simulink model "Complete_Model"  (R2015a)
settings: Solver=ode45  StartTime=0.0  StopTime=35  RelTol=1e-4
values from neighbouring files (symbols this model uses):
  g = 9.71    [Run_First.m]
undefined symbols (not defined in the file or in its folder): Earth, Receive, Send, WGS84
libraries: simulink x26, aerolibconvert2 x4, aerolibfltsims x3, aerolib6dof2 x1, aerolibnav x1, aerolibtransform2 x1, aerolibanimutils x1
settings Model: CovSFcnEnable=off  Creator=behill  LastModifiedBy=Bryce
settings DebuggingCC: AlgebraicLoopMsg=none  UnderspecifiedInitializationDetection=Classic  MergeDetectMultiDrivingBlocksExec=none

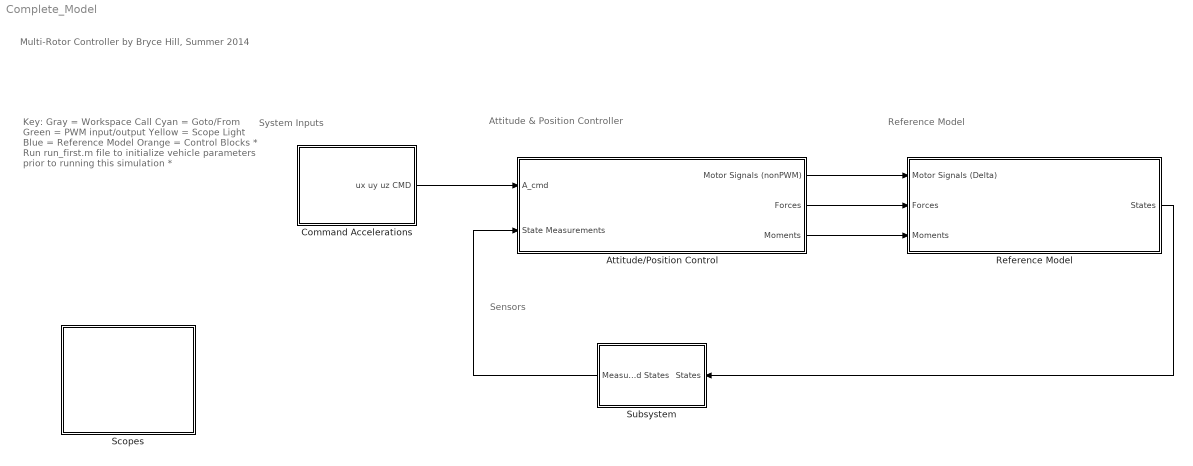
== system Complete_Model ==
  note: Sensors
  note: Reference Model
  note: Attitude & Position Controller
  note: System Inputs
  note: Multi-Rotor Controller
      | by Bryce Hill, Summer 2014
  note: Key:
      | Gray = Workspace Call
      | Cyan = Goto/From
      | Green = PWM input/output
      | Yellow = Scope
      | Light Blue = Reference Model
      | Orange = Control Blocks
      |
      | * Run run_first.m file to initialize vehicle parameters prior to running this simulation *
  Attitude/Position Control : Subsystem
  Command Accelerations : Subsystem
  Reference Model : Subsystem
  Scopes : Subsystem
  Subsystem : Subsystem
  wires:
  Command Accelerations/1(ux uy uz CMD) -> Attitude/Position Control/1(A_cmd)
  Attitude/Position Control/1(Motor Signals (nonPWM)) -> Reference Model/1(Motor Signals (Delta))
  Attitude/Position Control/2(Forces) -> Reference Model/2(Forces)
  Attitude/Position Control/3(Moments) -> Reference Model/3(Moments)
  Reference Model/1(States) -> Subsystem/1(States)
  Subsystem/1(Measured States) -> Attitude/Position Control/2(State Measurements)

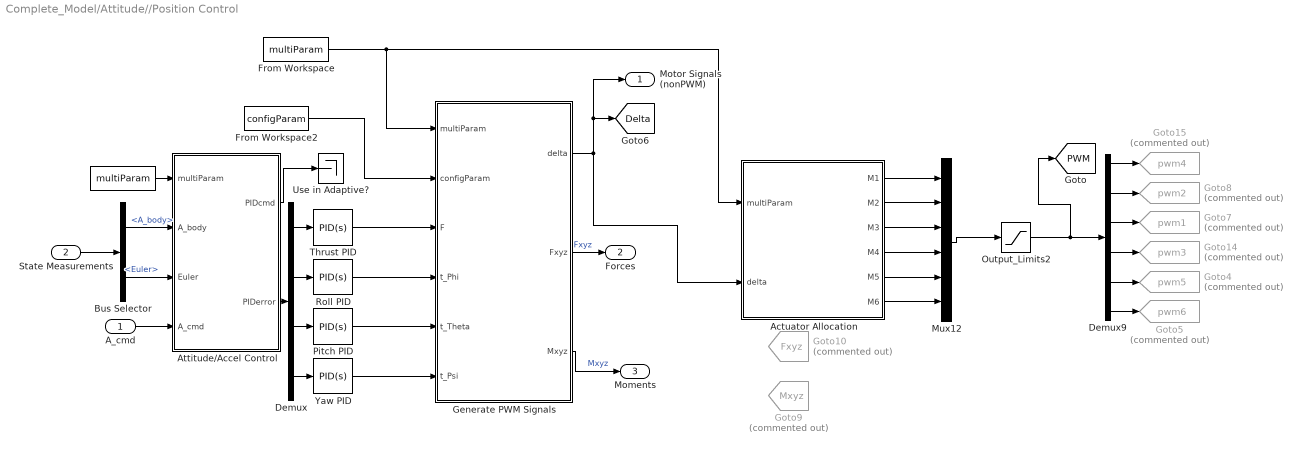
== system Complete_Model/Attitude//Position Control ==
  A_cmd : Inport
  State Measurements : Inport  Port=2
  " " : FromWorkspace  VariableName=multiParam  SampleTime=0
  Actuator Allocation : MATLAB Function  TreatAsAtomicUnit=on
  "Attitude/Accel Control " : MATLAB Function  TreatAsAtomicUnit=on
  Bus Selector : BusSelector  OutputSignals=A_body,Euler
  Demux : Demux
  Demux9 : Demux  Outputs=6
  From Workspace : FromWorkspace  VariableName=multiParam  SampleTime=0
  From Workspace2 : FromWorkspace  VariableName=configParam  SampleTime=0
  Generate PWM Signals : MATLAB Function  TreatAsAtomicUnit=on
  Goto10 : Goto  Commented=on  GotoTag=Fxyz  TagVisibility=global
  Goto14 : Goto  Commented=on  GotoTag=pwm3  TagVisibility=global
  Goto15 : Goto  Commented=on  GotoTag=pwm4  TagVisibility=global
  Goto4 : Goto  Commented=on  GotoTag=pwm5  TagVisibility=global
  Goto5 : Goto  Commented=on  GotoTag=pwm6  TagVisibility=global
  Goto7 : Goto  Commented=on  GotoTag=pwm1  TagVisibility=global
  Goto8 : Goto  Commented=on  GotoTag=pwm2  TagVisibility=global
  Goto9 : Goto  Commented=on  GotoTag=Mxyz  TagVisibility=global
  Mux12 : Mux  Inputs=6
  Output_Limits2 : Saturate  UpperLimit=2000  LowerLimit=1000
  Pitch PID : simulink/Continuous/PID Controller  Controller=PID  TimeDomain=Continuous-time  SampleTime=-1  IntegratorMethod=Forward Euler  FilterMethod=Forward Euler  Form=Parallel  UseFilter=on  ControllerParametersSource=internal  P=0.0917183656646997  I=0.00072113153908676  D=1.05906791895105  N=2.12291335792304  InitialConditionSource=internal  InitialConditionForIntegrator=0  InitialConditionForFilter=0  ExternalReset=none  LimitOutput=off  UpperSaturationLimit=inf  LowerSaturationLimit=-inf  LinearizeAsGain=on  AntiWindupMode=none  Kb=1  TrackingMode=off  Kt=1  PParamMin=[]  PParamMax=[]  IParamMin=[]  IParamMax=[]  DParamMin=[]  DParamMax=[]  NParamMin=[]  NParamMax=[]  KbParamMin=[]  KbParamMax=[]  KtParamMin=[]  KtParamMax=[]  POutMin=[]  POutMax=[]  IOutMin=[]  IOutMax=[]  DOutMin=[]  DOutMax=[]  NOutMin=[]  NOutMax=[]  KbOutMin=[]  KbOutMax=[]  KtOutMin=[]  KtOutMax=[]  IntegratorOutMin=[]  IntegratorOutMax=[]  FilterOutMin=[]  FilterOutMax=[]  SumOutMin=[]  SumOutMax=[]  SumI1OutMin=[]  SumI1OutMax=[]  SumI2OutMin=[]  SumI2OutMax=[]  SumI3OutMin=[]  SumI3OutMax=[]  SumDOutMin=[]  SumDOutMax=[]  SaturationOutMin=[]  SaturationOutMax=[]  IntegratorContinuousStateAttributes=''  IntegratorStateMustResolveToSignalObject=off  IntegratorRTWStateStorageClass=Auto  FilterContinuousStateAttributes=''  FilterStateMustResolveToSignalObject=off  FilterRTWStateStorageClass=Auto  DifferentiatorICPrevScaledInput=0  DifferentiatorOutMin=[]  DifferentiatorOutMax=[]
  Roll PID : simulink/Continuous/PID Controller  Controller=PID  TimeDomain=Continuous-time  SampleTime=-1  IntegratorMethod=Forward Euler  FilterMethod=Forward Euler  Form=Parallel  UseFilter=on  ControllerParametersSource=internal  P=0.231481505773178  I=0.0144568768471083  D=0.336499020225336  N=16.862900200716  InitialConditionSource=internal  InitialConditionForIntegrator=0  InitialConditionForFilter=0  ExternalReset=none  LimitOutput=off  UpperSaturationLimit=inf  LowerSaturationLimit=-inf  LinearizeAsGain=on  AntiWindupMode=none  Kb=1  TrackingMode=off  Kt=1  PParamMin=[]  PParamMax=[]  IParamMin=[]  IParamMax=[]  DParamMin=[]  DParamMax=[]  NParamMin=[]  NParamMax=[]  KbParamMin=[]  KbParamMax=[]  KtParamMin=[]  KtParamMax=[]  POutMin=[]  POutMax=[]  IOutMin=[]  IOutMax=[]  DOutMin=[]  DOutMax=[]  NOutMin=[]  NOutMax=[]  KbOutMin=[]  KbOutMax=[]  KtOutMin=[]  KtOutMax=[]  IntegratorOutMin=[]  IntegratorOutMax=[]  FilterOutMin=[]  FilterOutMax=[]  SumOutMin=[]  SumOutMax=[]  SumI1OutMin=[]  SumI1OutMax=[]  SumI2OutMin=[]  SumI2OutMax=[]  SumI3OutMin=[]  SumI3OutMax=[]  SumDOutMin=[]  SumDOutMax=[]  SaturationOutMin=[]  SaturationOutMax=[]  IntegratorContinuousStateAttributes=''  IntegratorStateMustResolveToSignalObject=off  IntegratorRTWStateStorageClass=Auto  FilterContinuousStateAttributes=''  FilterStateMustResolveToSignalObject=off  FilterRTWStateStorageClass=Auto  DifferentiatorICPrevScaledInput=0  DifferentiatorOutMin=[]  DifferentiatorOutMax=[]
  Thrust PID : simulink/Continuous/PID Controller  Controller=PID  TimeDomain=Continuous-time  SampleTime=-1  IntegratorMethod=Forward Euler  FilterMethod=Forward Euler  Form=Parallel  UseFilter=on  ControllerParametersSource=internal  P=10  I=10  D=15  N=100  InitialConditionSource=internal  InitialConditionForIntegrator=0  InitialConditionForFilter=0  ExternalReset=none  LimitOutput=off  UpperSaturationLimit=inf  LowerSaturationLimit=-inf  LinearizeAsGain=on  AntiWindupMode=none  Kb=1  TrackingMode=off  Kt=1  PParamMin=[]  PParamMax=[]  IParamMin=[]  IParamMax=[]  DParamMin=[]  DParamMax=[]  NParamMin=[]  NParamMax=[]  KbParamMin=[]  KbParamMax=[]  KtParamMin=[]  KtParamMax=[]  POutMin=[]  POutMax=[]  IOutMin=[]  IOutMax=[]  DOutMin=[]  DOutMax=[]  NOutMin=[]  NOutMax=[]  KbOutMin=[]  KbOutMax=[]  KtOutMin=[]  KtOutMax=[]  IntegratorOutMin=[]  IntegratorOutMax=[]  FilterOutMin=[]  FilterOutMax=[]  SumOutMin=[]  SumOutMax=[]  SumI1OutMin=[]  SumI1OutMax=[]  SumI2OutMin=[]  SumI2OutMax=[]  SumI3OutMin=[]  SumI3OutMax=[]  SumDOutMin=[]  SumDOutMax=[]  SaturationOutMin=[]  SaturationOutMax=[]  IntegratorContinuousStateAttributes=''  IntegratorStateMustResolveToSignalObject=off  IntegratorRTWStateStorageClass=Auto  FilterContinuousStateAttributes=''  FilterStateMustResolveToSignalObject=off  FilterRTWStateStorageClass=Auto  DifferentiatorICPrevScaledInput=0  DifferentiatorOutMin=[]  DifferentiatorOutMax=[]
  Use in Adaptive? : Terminator
  Yaw PID : simulink/Continuous/PID Controller  Controller=PID  TimeDomain=Continuous-time  SampleTime=-1  IntegratorMethod=Forward Euler  FilterMethod=Forward Euler  Form=Parallel  UseFilter=on  ControllerParametersSource=internal  P=0.00458591828325413  I=3.60565769544884e-05  D=0.0529533959477758  N=2.12291335792304  InitialConditionSource=internal  InitialConditionForIntegrator=0  InitialConditionForFilter=0  ExternalReset=none  LimitOutput=off  UpperSaturationLimit=inf  LowerSaturationLimit=-inf  LinearizeAsGain=on  AntiWindupMode=none  Kb=1  TrackingMode=off  Kt=1  PParamMin=[]  PParamMax=[]  IParamMin=[]  IParamMax=[]  DParamMin=[]  DParamMax=[]  NParamMin=[]  NParamMax=[]  KbParamMin=[]  KbParamMax=[]  KtParamMin=[]  KtParamMax=[]  POutMin=[]  POutMax=[]  IOutMin=[]  IOutMax=[]  DOutMin=[]  DOutMax=[]  NOutMin=[]  NOutMax=[]  KbOutMin=[]  KbOutMax=[]  KtOutMin=[]  KtOutMax=[]  IntegratorOutMin=[]  IntegratorOutMax=[]  FilterOutMin=[]  FilterOutMax=[]  SumOutMin=[]  SumOutMax=[]  SumI1OutMin=[]  SumI1OutMax=[]  SumI2OutMin=[]  SumI2OutMax=[]  SumI3OutMin=[]  SumI3OutMax=[]  SumDOutMin=[]  SumDOutMax=[]  SaturationOutMin=[]  SaturationOutMax=[]  IntegratorContinuousStateAttributes=''  IntegratorStateMustResolveToSignalObject=off  IntegratorRTWStateStorageClass=Auto  FilterContinuousStateAttributes=''  FilterStateMustResolveToSignalObject=off  FilterRTWStateStorageClass=Auto  DifferentiatorICPrevScaledInput=0  DifferentiatorOutMin=[]  DifferentiatorOutMax=[]
  Motor Signals (nonPWM) : Outport
  Forces : Outport  Port=2
  Moments : Outport  Port=3
  tag scope: Delta=global, PWM=global
  wires:
  Yaw PID/1 -> Generate PWM Signals/6(t_Psi)
  Thrust PID/1 -> Generate PWM Signals/3(F)
  Pitch PID/1 -> Generate PWM Signals/5(t_Theta)
  Roll PID/1 -> Generate PWM Signals/4(t_Phi)
  " "/1 -> "Attitude/Accel Control "/1(multiParam)
  "Attitude/Accel Control "/1(PIDcmd) -> Use in Adaptive?/1
  "Attitude/Accel Control "/2(PIDerror) -> Demux/1
  Demux/1 -> Thrust PID/1
  Actuator Allocation/4(M4) -> Mux12/4
  Demux9/5 -> Goto4/1
  Demux9/6 -> Goto5/1
  Actuator Allocation/3(M3) -> Mux12/3
  Actuator Allocation/1(M1) -> Mux12/1
  Demux9/1 -> Goto15/1
  Demux9/2 -> Goto8/1
  Demux9/3 -> Goto7/1
  Demux9/4 -> Goto14/1
  Mux12/1 -> Output_Limits2/1
  Demux/2 -> Roll PID/1
  Demux/4 -> Yaw PID/1
  Generate PWM Signals/1(delta) -> [Delta], Motor Signals (nonPWM)/1, Actuator Allocation/2(delta)
  Demux/3 -> Pitch PID/1
  Actuator Allocation/2(M2) -> Mux12/2
  Generate PWM Signals/2(Fxyz) -> Forces/1  "Fxyz"
  A_cmd/1 -> "Attitude/Accel Control "/4(A_cmd)
  Generate PWM Signals/3(Mxyz) -> Moments/1  "Mxyz"
  Bus Selector/1 -> "Attitude/Accel Control "/2(A_body)  "<A_body>"
  Bus Selector/2 -> "Attitude/Accel Control "/3(Euler)  "<Euler>"
  State Measurements/1 -> Bus Selector/1
  From Workspace/1 -> Actuator Allocation/1(multiParam), Generate PWM Signals/1(multiParam)
  From Workspace2/1 -> Generate PWM Signals/2(configParam)
  Output_Limits2/1 -> Demux9/1, [PWM]
  Actuator Allocation/5(M5) -> Mux12/5
  Actuator Allocation/6(M6) -> Mux12/6

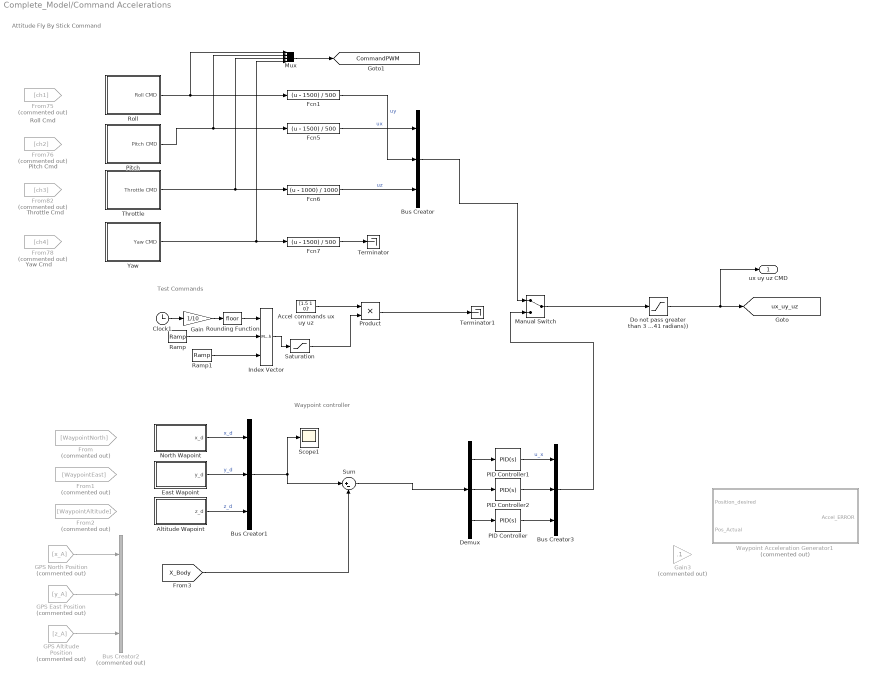
== system Complete_Model/Command Accelerations ==
  note: Waypoint controller
  note: Test Commands
  note: Attitude Fly By Stick Command
  note: Roll Cmd
  note: Throttle Cmd
  note: Yaw Cmd
  note: Pitch Cmd
  Accel commands ux uy uz : Constant  Value=[1.5 1 0]'
  Altitude Wapoint : Subsystem
  Bus Creator : BusCreator  Inputs=3
  Bus Creator1 : BusCreator  Inputs=3
  Bus Creator2 : BusCreator  Commented=on  Inputs=3
  Bus Creator3 : BusCreator  Inputs=3
  Clock1 : Clock
  Demux : Demux  Outputs=3
  Do not pass greater than 3 m/s (23 degrees (.41 radians)) : Saturate  UpperLimit=1  LowerLimit=-1
  East Wapoint : Subsystem
  Fcn1 : Fcn  Expr=(u - 1500) / 500
  Fcn5 : Fcn  Expr=(u - 1500) / 500
  Fcn6 : Fcn  Expr=(u - 1000) / 1000
  Fcn7 : Fcn  Expr=(u - 1500) / 500
  From : From  Commented=on  GotoTag=WaypointNorth
  From1 : From  Commented=on  GotoTag=WaypointEast
  From2 : From  Commented=on  GotoTag=WaypointAltitude
  From75 : From  Commented=on  GotoTag=ch1
  From76 : From  Commented=on  GotoTag=ch2
  From78 : From  Commented=on  GotoTag=ch4
  From82 : From  Commented=on  GotoTag=ch3
  GPS Altitude Position : From  Commented=on  GotoTag=z_A
  GPS East Position : From  Commented=on  GotoTag=y_A
  GPS North Position : From  Commented=on  GotoTag=x_A
  Gain : Gain  Gain=1/10
  Gain3 : Gain  Commented=on  Gain=.1
  Index Vector : MultiPortSwitch  DataPortOrder=Zero-based contiguous  Inputs=2  DiagnosticForDefault=None  zeroidx=on
  Manual Switch : ManualSwitch
  Mux : Mux
  North Wapoint : Subsystem
  PID Controller : simulink/Continuous/PID Controller  Controller=PID  TimeDomain=Continuous-time  SampleTime=-1  IntegratorMethod=Forward Euler  FilterMethod=Forward Euler  Form=Parallel  UseFilter=on  ControllerParametersSource=internal  P=0.00117950118646568  I=9.51975576620891e-07  D=0.104202467385276  N=0.212291335792304  InitialConditionSource=internal  InitialConditionForIntegrator=0  InitialConditionForFilter=0  ExternalReset=none  LimitOutput=off  UpperSaturationLimit=inf  LowerSaturationLimit=-inf  LinearizeAsGain=on  AntiWindupMode=none  Kb=1  TrackingMode=off  Kt=1  PParamMin=[]  PParamMax=[]  IParamMin=[]  IParamMax=[]  DParamMin=[]  DParamMax=[]  NParamMin=[]  NParamMax=[]  KbParamMin=[]  KbParamMax=[]  KtParamMin=[]  KtParamMax=[]  POutMin=[]  POutMax=[]  IOutMin=[]  IOutMax=[]  DOutMin=[]  DOutMax=[]  NOutMin=[]  NOutMax=[]  KbOutMin=[]  KbOutMax=[]  KtOutMin=[]  KtOutMax=[]  IntegratorOutMin=[]  IntegratorOutMax=[]  FilterOutMin=[]  FilterOutMax=[]  SumOutMin=[]  SumOutMax=[]  SumI1OutMin=[]  SumI1OutMax=[]  SumI2OutMin=[]  SumI2OutMax=[]  SumI3OutMin=[]  SumI3OutMax=[]  SumDOutMin=[]  SumDOutMax=[]  SaturationOutMin=[]  SaturationOutMax=[]  IntegratorContinuousStateAttributes=''  IntegratorStateMustResolveToSignalObject=off  IntegratorRTWStateStorageClass=Auto  FilterContinuousStateAttributes=''  FilterStateMustResolveToSignalObject=off  FilterRTWStateStorageClass=Auto  DifferentiatorICPrevScaledInput=0  DifferentiatorOutMin=[]  DifferentiatorOutMax=[]
  PID Controller1 : simulink/Continuous/PID Controller  Controller=PID  TimeDomain=Continuous-time  SampleTime=-1  IntegratorMethod=Forward Euler  FilterMethod=Forward Euler  Form=Parallel  UseFilter=on  ControllerParametersSource=internal  P=8.76810575019982e-09  I=2.11533755573293e-14  D=0.000329957020406041  N=0.000651400313625064  InitialConditionSource=internal  InitialConditionForIntegrator=0  InitialConditionForFilter=0  ExternalReset=none  LimitOutput=off  UpperSaturationLimit=inf  LowerSaturationLimit=-inf  LinearizeAsGain=on  AntiWindupMode=none  Kb=1  TrackingMode=off  Kt=1  PParamMin=[]  PParamMax=[]  IParamMin=[]  IParamMax=[]  DParamMin=[]  DParamMax=[]  NParamMin=[]  NParamMax=[]  KbParamMin=[]  KbParamMax=[]  KtParamMin=[]  KtParamMax=[]  POutMin=[]  POutMax=[]  IOutMin=[]  IOutMax=[]  DOutMin=[]  DOutMax=[]  NOutMin=[]  NOutMax=[]  KbOutMin=[]  KbOutMax=[]  KtOutMin=[]  KtOutMax=[]  IntegratorOutMin=[]  IntegratorOutMax=[]  FilterOutMin=[]  FilterOutMax=[]  SumOutMin=[]  SumOutMax=[]  SumI1OutMin=[]  SumI1OutMax=[]  SumI2OutMin=[]  SumI2OutMax=[]  SumI3OutMin=[]  SumI3OutMax=[]  SumDOutMin=[]  SumDOutMax=[]  SaturationOutMin=[]  SaturationOutMax=[]  IntegratorContinuousStateAttributes=''  IntegratorStateMustResolveToSignalObject=off  IntegratorRTWStateStorageClass=Auto  FilterContinuousStateAttributes=''  FilterStateMustResolveToSignalObject=off  FilterRTWStateStorageClass=Auto  DifferentiatorICPrevScaledInput=0  DifferentiatorOutMin=[]  DifferentiatorOutMax=[]
  PID Controller2 : simulink/Continuous/PID Controller  Controller=PID  TimeDomain=Continuous-time  SampleTime=-1  IntegratorMethod=Forward Euler  FilterMethod=Forward Euler  Form=Parallel  UseFilter=on  ControllerParametersSource=internal  P=0.345806907293553  I=0.007128817123713  D=3.36644459456349  N=372.899120284162  InitialConditionSource=internal  InitialConditionForIntegrator=0  InitialConditionForFilter=0  ExternalReset=none  LimitOutput=off  UpperSaturationLimit=inf  LowerSaturationLimit=-inf  LinearizeAsGain=on  AntiWindupMode=none  Kb=1  TrackingMode=off  Kt=1  PParamMin=[]  PParamMax=[]  IParamMin=[]  IParamMax=[]  DParamMin=[]  DParamMax=[]  NParamMin=[]  NParamMax=[]  KbParamMin=[]  KbParamMax=[]  KtParamMin=[]  KtParamMax=[]  POutMin=[]  POutMax=[]  IOutMin=[]  IOutMax=[]  DOutMin=[]  DOutMax=[]  NOutMin=[]  NOutMax=[]  KbOutMin=[]  KbOutMax=[]  KtOutMin=[]  KtOutMax=[]  IntegratorOutMin=[]  IntegratorOutMax=[]  FilterOutMin=[]  FilterOutMax=[]  SumOutMin=[]  SumOutMax=[]  SumI1OutMin=[]  SumI1OutMax=[]  SumI2OutMin=[]  SumI2OutMax=[]  SumI3OutMin=[]  SumI3OutMax=[]  SumDOutMin=[]  SumDOutMax=[]  SaturationOutMin=[]  SaturationOutMax=[]  IntegratorContinuousStateAttributes=''  IntegratorStateMustResolveToSignalObject=off  IntegratorRTWStateStorageClass=Auto  FilterContinuousStateAttributes=''  FilterStateMustResolveToSignalObject=off  FilterRTWStateStorageClass=Auto  DifferentiatorICPrevScaledInput=0  DifferentiatorOutMin=[]  DifferentiatorOutMax=[]
  Pitch : Subsystem
  Product : Product
  Ramp : simulink/Sources/Ramp  slope=5/5  start=0  X0=0
  Ramp1 : simulink/Sources/Ramp  slope=-2  start=10  X0=5
  Roll : Subsystem
  Rounding Function : Rounding
  Saturation : Saturate  UpperLimit=5  LowerLimit=-5
  Scope1 : Scope
      settings: ShowLegends=on  YMin=0  YMax=10  SaveName=ScopeData8
  Sum : Sum  Inputs=|+-
  Terminator : Terminator
  Terminator1 : Terminator
  Throttle : Subsystem
  Waypoint Acceleration Generator1 : MATLAB Function  Commented=on  TreatAsAtomicUnit=on
  Yaw : Subsystem
  ux uy uz CMD : Outport
  tag scope: CommandPWM=global, ux_uy_uz=global
  wires:
  Fcn7/1 -> Terminator/1
  Mux/1 -> [CommandPWM]
  Fcn6/1 -> Bus Creator/3  "uz"
  Fcn5/1 -> Bus Creator/1  "ux"
  Fcn1/1 -> Bus Creator/2  "uy"
  Bus Creator/1 -> Manual Switch/1
  Roll/1(Roll CMD) -> Mux/1, Fcn1/1
  Pitch/1(Pitch CMD) -> Mux/2, Fcn5/1
  Yaw/1(Yaw CMD) -> Mux/4, Fcn7/1
  Throttle/1(Throttle CMD) -> Fcn6/1, Mux/3
  Saturation/1 -> Product/2
  Rounding Function/1 -> Index Vector/1
  Product/1 -> Terminator1/1
  Accel commands ux uy uz/1 -> Product/1
  Ramp1/1 -> Index Vector/3
  Ramp/1 -> Index Vector/2
  Clock1/1 -> Gain/1
  Index Vector/1 -> Saturation/1
  Gain/1 -> Rounding Function/1
  Manual Switch/1 -> Do not pass greater than 3 m/s (23 degrees (.41 radians))/1
  Do not pass greater than 3 m/s (23 degrees (.41 radians))/1 -> ux uy uz CMD/1, [ux_uy_uz]
  North Wapoint/1(x_d) -> Bus Creator1/1  "x_d"
  East Wapoint/1(y_d) -> Bus Creator1/2  "y_d"
  Altitude Wapoint/1(z_d) -> Bus Creator1/3  "z_d"
  Bus Creator1/1 -> Sum/1, Scope1/1
  [X_Body] -> Sum/2
  GPS North Position/1 -> Bus Creator2/1
  GPS East Position/1 -> Bus Creator2/2
  GPS Altitude Position/1 -> Bus Creator2/3
  Sum/1 -> Demux/1
  Demux/2 -> PID Controller2/1
  PID Controller1/1 -> Bus Creator3/1  "u_x"
  Bus Creator3/1 -> Manual Switch/2
  Demux/3 -> PID Controller/1
  PID Controller/1 -> Bus Creator3/3
  Demux/1 -> PID Controller1/1
  PID Controller2/1 -> Bus Creator3/2

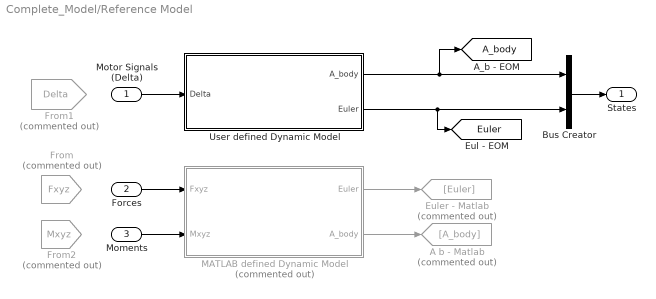
== system Complete_Model/Reference Model ==
  Motor Signals (Delta) : Inport
  Forces : Inport  Port=2
  Moments : Inport  Port=3
  A b - Matlab : Goto  Commented=on  GotoTag=A_body
  Bus Creator : BusCreator  Inputs=2
  Euler - Matlab : Goto  Commented=on  GotoTag=Euler
  From : From  Commented=on  GotoTag=Fxyz  TagVisibility=global
  From1 : From  Commented=on  GotoTag=Delta  TagVisibility=global
  From2 : From  Commented=on  GotoTag=Mxyz  TagVisibility=global
  MATLAB defined Dynamic Model : Subsystem  Commented=on
  User defined Dynamic Model : Subsystem
  States : Outport
  tag scope: A_body=global, Euler=global
  wires:
  MATLAB defined Dynamic Model/1(Euler) -> Euler - Matlab/1
  MATLAB defined Dynamic Model/2(A_body) -> A b - Matlab/1
  Motor Signals (Delta)/1 -> User defined Dynamic Model/1(Delta)
  Forces/1 -> MATLAB defined Dynamic Model/1(Fxyz)
  Moments/1 -> MATLAB defined Dynamic Model/2(Mxyz)
  User defined Dynamic Model/1(A_body) -> [A_body], Bus Creator/1
  User defined Dynamic Model/2(Euler) -> Bus Creator/2, [Euler]
  Bus Creator/1 -> States/1

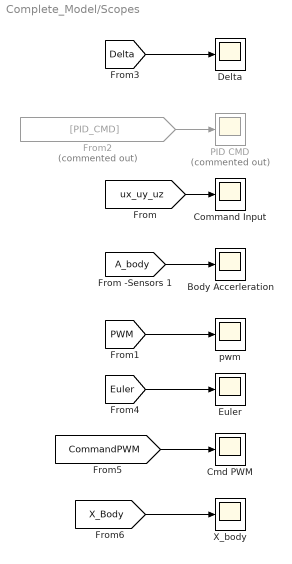
== system Complete_Model/Scopes ==
  Body Accerleration : Scope
      settings: ShowLegends=on  YMin=-1.3  YMax=0.7  SaveName=ScopeData2
  Cmd PWM : Scope
      settings: TimeRange=35  YMin=1500  YMax=1521  SaveName=ScopeData4
  Command Input : Scope
      settings: ShowLegends=on  YMin=-0.25  YMax=0.2  SaveName=ScopeData3
  Delta : Scope
      settings: YMin=27.5  YMax=33
  Euler : Scope
      settings: YMin=-2.75e-07  YMax=2.5e-08  SaveName=ScopeData6
  From2 : From  Commented=on  GotoTag=PID_CMD
  PID CMD : Scope  Commented=on
  X_body : Scope
      settings: ShowLegends=on  YMin=-10  YMax=190  SaveName=ScopeData9
  pwm : Scope
      settings: YMin=1463  YMax=1479  SaveName=ScopeData5
  wires:
  [ux_uy_uz] -> Command Input/1
  [PWM] -> pwm/1
  [A_body] -> Body Accerleration/1
  [Delta] -> Delta/1
  From2/1 -> PID CMD/1
  [Euler] -> Euler/1
  [CommandPWM] -> Cmd PWM/1
  [X_Body] -> X_body/1

== system Complete_Model/Subsystem ==
  States : Inport
  Measured States : Outport
  wires:
  States/1 -> Measured States/1

== system Complete_Model/Command Accelerations/Altitude Wapoint ==
  Clock : Clock
  Constant : Constant  Value=-10
  Constant1 : Constant  Value=10
  Switch : Switch  Criteria=u2 > Threshold  Threshold=30
  z_d : Outport
  wires:
  Clock/1 -> Switch/2
  Constant1/1 -> Switch/3
  Constant/1 -> z_d/1

== system Complete_Model/Command Accelerations/East Wapoint ==
  Clock : Clock
  Constant : Constant  Value=0
  Constant1 : Constant  Value=.01
  Switch : Switch  Criteria=u2 > Threshold  Threshold=30
  y_d : Outport
  wires:
  Clock/1 -> Switch/2
  Constant1/1 -> Switch/3
  Constant/1 -> y_d/1

== system Complete_Model/Command Accelerations/North Wapoint ==
  Clock : Clock
  Constant : Constant  Value=10
  Constant1 : Constant  Value=5
  Switch : Switch  Criteria=u2 > Threshold  Threshold=30
  x_d : Outport
  wires:
  Clock/1 -> Switch/2
  Constant1/1 -> Switch/3
  Constant/1 -> x_d/1

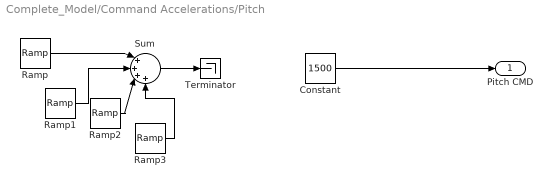
== system Complete_Model/Command Accelerations/Pitch ==
  Constant : Constant  Value=1500
  Ramp : simulink/Sources/Ramp  slope=10  start=5  X0=250
  Ramp1 : simulink/Sources/Ramp  slope=-10  start=10  X0=300
  Ramp2 : simulink/Sources/Ramp  slope=-10  start=15  X0=300
  Ramp3 : simulink/Sources/Ramp  slope=10  start=20  X0=250
  Sum : Sum  Inputs=|++++
  Terminator : Terminator
  Pitch CMD : Outport
  wires:
  Ramp/1 -> Sum/1
  Ramp1/1 -> Sum/2
  Ramp2/1 -> Sum/3
  Ramp3/1 -> Sum/4
  Sum/1 -> Terminator/1
  Constant/1 -> Pitch CMD/1

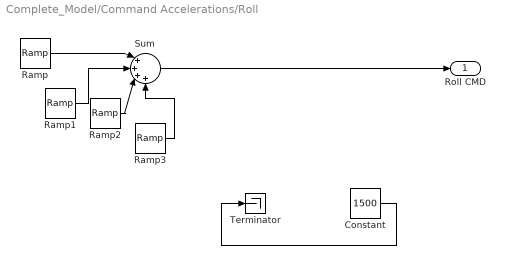
== system Complete_Model/Command Accelerations/Roll ==
  Constant : Constant  Value=1500
  Ramp : simulink/Sources/Ramp  slope=10  start=5  X0=350
  Ramp1 : simulink/Sources/Ramp  slope=-10  start=10  X0=400
  Ramp2 : simulink/Sources/Ramp  slope=-10  start=15  X0=400
  Ramp3 : simulink/Sources/Ramp  slope=10  start=20  X0=350
  Sum : Sum  Inputs=|++++
  Terminator : Terminator
  Roll CMD : Outport
  wires:
  Ramp/1 -> Sum/1
  Ramp1/1 -> Sum/2
  Ramp2/1 -> Sum/3
  Ramp3/1 -> Sum/4
  Constant/1 -> Terminator/1
  Sum/1 -> Roll CMD/1

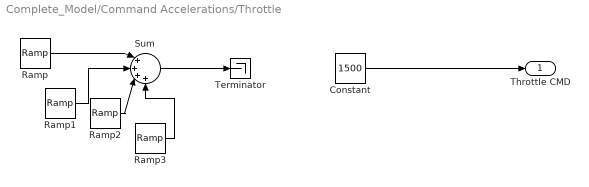
== system Complete_Model/Command Accelerations/Throttle ==
  Constant : Constant  Value=1500
  Ramp : simulink/Sources/Ramp  slope=10  start=5  X0=250
  Ramp1 : simulink/Sources/Ramp  slope=-10  start=10  X0=300
  Ramp2 : simulink/Sources/Ramp  slope=-10  start=15  X0=300
  Ramp3 : simulink/Sources/Ramp  slope=10  start=20  X0=250
  Sum : Sum  Inputs=|++++
  Terminator : Terminator
  Throttle CMD : Outport
  wires:
  Ramp/1 -> Sum/1
  Ramp1/1 -> Sum/2
  Ramp2/1 -> Sum/3
  Ramp3/1 -> Sum/4
  Sum/1 -> Terminator/1
  Constant/1 -> Throttle CMD/1

== system Complete_Model/Command Accelerations/Yaw ==
  Constant : Constant  Value=1500
  Ramp : simulink/Sources/Ramp  slope=10  start=5  X0=250
  Ramp1 : simulink/Sources/Ramp  slope=-10  start=10  X0=300
  Ramp2 : simulink/Sources/Ramp  slope=-10  start=15  X0=300
  Ramp3 : simulink/Sources/Ramp  slope=10  start=20  X0=250
  Sum : Sum  Inputs=|++++
  Terminator : Terminator
  Yaw CMD : Outport
  wires:
  Ramp/1 -> Sum/1
  Ramp1/1 -> Sum/2
  Ramp2/1 -> Sum/3
  Ramp3/1 -> Sum/4
  Constant/1 -> Yaw CMD/1
  Sum/1 -> Terminator/1

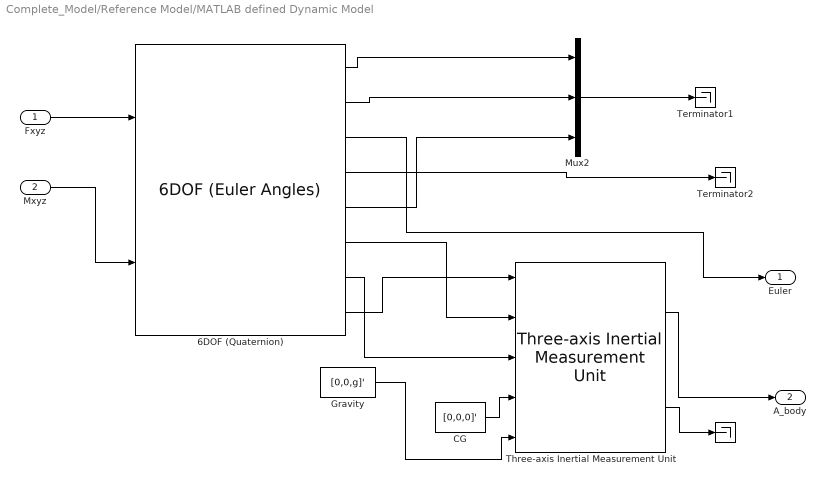
== system Complete_Model/Reference Model/MATLAB defined Dynamic Model ==
  Fxyz : Inport
  Mxyz : Inport  Port=2
  " " : Terminator
  6DOF (Quaternion) : aerolib6dof2/6DOF (Euler Angles)  units=Metric (MKS)  mtype=Fixed  rep=Quaternion  xme_0=[0 0 0]  Vm_0=[0 0 0]  eul_0=[0 0 0]  pm_0=[0 0 0]  mass_0=2.4  mass_e=0.5  mass_f=2.0  inertia=[.05,0,0;0,.05,0;0,0,.05]  inertia_e=eye(3)  inertia_f=2*eye(3)  k_quat=1.0  vre_flag=on
  CG : Constant  Value=[0,0,0]'
  Gravity : Constant  Value=[0,0,g]'
  Mux2 : Mux  Inputs=3
  Terminator1 : Terminator
  Terminator2 : Terminator
  Three-axis Inertial Measurement Unit : aerolibnav/Three-axis Inertial Measurement Unit  units=Metric (MKS)  imu=[0 0 0]  dtype_a=on  w_a=190  z_a=0.707  a_sf_cc=[1 0 0; 0 1 0; 0 0 1]  a_bias=[0 0 0]  a_sat="[-inf  -inf  -inf  inf inf inf]"  dtype_g=on  w_g=190  z_g=0.707  g_sf_cc=[1 0 0; 0 1 0; 0 0 1]  g_bias=[0 0 0]  g_sens=[0 0 0]  g_sat="[-inf  -inf  -inf  inf inf inf]"  i_rand=on  i_seeds=[23093 23094 23095 23096 23097 23098]  i_pow=[0.001 0.001 0.001 0.0001 0.0001 0.0001]  i_Ts=0
  Euler : Outport
  A_body : Outport  Port=2
  wires:
  Mux2/1 -> Terminator1/1
  6DOF (Quaternion)/5 -> Mux2/3
  6DOF (Quaternion)/1 -> Mux2/1
  6DOF (Quaternion)/2 -> Mux2/2
  6DOF (Quaternion)/4 -> Terminator2/1
  6DOF (Quaternion)/8 -> Three-axis Inertial Measurement Unit/1
  6DOF (Quaternion)/6 -> Three-axis Inertial Measurement Unit/2
  6DOF (Quaternion)/7 -> Three-axis Inertial Measurement Unit/3
  Mxyz/1 -> 6DOF (Quaternion)/2
  6DOF (Quaternion)/3 -> Euler/1
  Fxyz/1 -> 6DOF (Quaternion)/1
  CG/1 -> Three-axis Inertial Measurement Unit/4
  Three-axis Inertial Measurement Unit/2 -> " "/1
  Gravity/1 -> Three-axis Inertial Measurement Unit/5
  Three-axis Inertial Measurement Unit/1 -> A_body/1

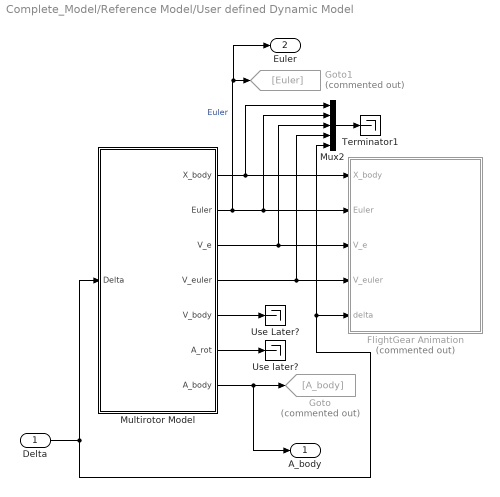
== system Complete_Model/Reference Model/User defined Dynamic Model ==
  Delta : Inport
  FlightGear Animation : Subsystem  Commented=on
  Goto : Goto  Commented=on  GotoTag=A_body
  Goto1 : Goto  Commented=on  GotoTag=Euler
  "Multirotor Model " : Subsystem
  Mux2 : Mux  Inputs=5
  Terminator1 : Terminator
  "Use Later? " : Terminator
  Use later? : Terminator
  A_body : Outport
  Euler : Outport  Port=2
  wires:
  Delta/1 -> "Multirotor Model "/1("Delta "), FlightGear Animation/5(delta), Mux2/5
  "Multirotor Model "/3(V_e) -> FlightGear Animation/3(V_e), Mux2/3
  "Multirotor Model "/6(A_rot) -> Use later?/1
  "Multirotor Model "/4(V_euler) -> FlightGear Animation/4(V_euler), Mux2/4
  Mux2/1 -> Terminator1/1
  "Multirotor Model "/5(V_body) -> "Use Later? "/1
  "Multirotor Model "/1(X_body) -> FlightGear Animation/1(X_body), Mux2/1
  "Multirotor Model "/2(Euler) -> FlightGear Animation/2(Euler), Mux2/2, Euler/1, Goto1/1  "Euler"
  "Multirotor Model "/7(A_body) -> A_body/1, Goto/1

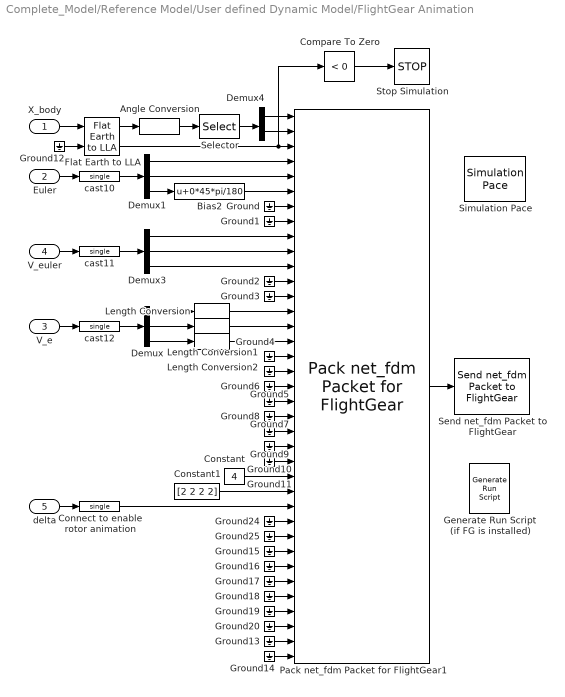
== system Complete_Model/Reference Model/User defined Dynamic Model/FlightGear Animation ==
  X_body : Inport
  Euler : Inport  Port=2
  V_e : Inport  Port=3
  V_euler : Inport  Port=4
  delta : Inport  Port=5
  Angle Conversion : aerolibconvert2/Angle Conversion  IU=deg  OU=rad
  Bias2 : Bias  Bias=0*45*pi/180
  Compare To Zero : simulink/Logic and Bit Operations/Compare To Zero  relop=<  OutDataTypeStr=boolean
  Connect to enable rotor animation : DataTypeConversion  OutDataTypeStr=single  SaturateOnIntegerOverflow=on
  Constant : Constant  Value=4  OutDataTypeStr=uint32
  Constant1 : Constant  Value=[2 2 2 2]  OutDataTypeStr=uint32
  Demux : Demux  Outputs=3
  Demux1 : Demux  Outputs=3
  Demux3 : Demux  Outputs=3
  Demux4 : Demux  Outputs=2
  Flat Earth to LLA : aerolibtransform2/Flat Earth to LLA  units=Metric (MKS)  ptype=Earth (WGS84)  F=1/298.257223563  R=6378137  LL0=[37.613553 -122.357195]  psi=0
  Generate Run Script (if FG is installed) : aerolibfltsims/Generate Run Script  OutputFileName=runfg.bat  FlightGearBaseDirectory=C:\Program Files\FlightGear  GeometryModelName=arducopter  DestinationPort=5502  OriginAddress=172.16.33.216  OriginPort=5505  LocalAddress=172.16.33.216  AirportId=KSFO  RunwayId=10L  InitialAltitude=0  InitialHeading=0  OffsetDistance=0  OffsetAzimuth=0  GenerateFile=off  Architecture=Default  dataFlow=Send-Receive
  Ground{,1..20,24..25} (23 alike) : Ground
  Length Conversion : aerolibconvert2/Length Conversion  IU=m  OU=ft
  Length Conversion1 : aerolibconvert2/Length Conversion  IU=m  OU=ft
  Length Conversion2 : aerolibconvert2/Length Conversion  IU=m  OU=ft
  Pack net_fdm Packet for FlightGear1 : aerolibfltsims/Pack net_fdm Packet for FlightGear  FlightGearVersion=v2.8  ShowPositionAttitudeInputs=on  ShowVelocityAccelerationInputs=on  ShowControlSurfacePositionInputs=off  ShowEngineFuelInputs=on  ShowLandingGearInputs=off  ShowEnvironmentInputs=off  SampleTime=1/30
  Selector : Selector  InputPortWidth=2  Indices=[2 1]
  Send net_fdm Packet to FlightGear : aerolibfltsims/Send net_fdm Packet to FlightGear  DestinationIpAddress=172.16.33.216  DestinationPort=5502  LocalIpPort=-1  varLen=off  SampleTime=1/30
  Simulation Pace : aerolibanimutils/Simulation Pace  SimulationPace=1  SleepMode=MATLAB Thread  OutputPaceError=off  SampleTime=1/30
      settings: AttributesFormatString=%<SimulationPace> sec/sec
  Stop Simulation : Stop
  cast10 : DataTypeConversion  OutDataTypeStr=single  SaturateOnIntegerOverflow=on
  cast11 : DataTypeConversion  OutDataTypeStr=single  SaturateOnIntegerOverflow=on
  cast12 : DataTypeConversion  OutDataTypeStr=single  SaturateOnIntegerOverflow=on
  wires:
  Demux/1 -> Length Conversion/1
  Demux/2 -> Length Conversion1/1
  Demux/3 -> Length Conversion2/1
  Ground/1 -> Pack net_fdm Packet for FlightGear1/7
  V_euler/1 -> cast11/1
  Ground7/1 -> Pack net_fdm Packet for FlightGear1/20
  Ground2/1 -> Pack net_fdm Packet for FlightGear1/12
  Ground9/1 -> Pack net_fdm Packet for FlightGear1/22
  Ground10/1 -> Pack net_fdm Packet for FlightGear1/23
  Ground5/1 -> Pack net_fdm Packet for FlightGear1/18
  Ground11/1 -> Pack net_fdm Packet for FlightGear1/24
  Ground4/1 -> Pack net_fdm Packet for FlightGear1/17
  Ground8/1 -> Pack net_fdm Packet for FlightGear1/21
  Ground1/1 -> Pack net_fdm Packet for FlightGear1/8
  Ground3/1 -> Pack net_fdm Packet for FlightGear1/13
  Ground6/1 -> Pack net_fdm Packet for FlightGear1/19
  Demux3/1 -> Pack net_fdm Packet for FlightGear1/9
  Demux1/3 -> Bias2/1
  Demux1/2 -> Pack net_fdm Packet for FlightGear1/5
  Demux1/1 -> Pack net_fdm Packet for FlightGear1/4
  Demux3/2 -> Pack net_fdm Packet for FlightGear1/10
  Demux3/3 -> Pack net_fdm Packet for FlightGear1/11
  Pack net_fdm Packet for FlightGear1/1 -> Send net_fdm Packet to FlightGear/1
  Euler/1 -> cast10/1
  cast11/1 -> Demux3/1
  cast10/1 -> Demux1/1
  cast12/1 -> Demux/1
  Flat Earth to LLA/1 -> Angle Conversion/1
  Demux4/1 -> Pack net_fdm Packet for FlightGear1/1
  Demux4/2 -> Pack net_fdm Packet for FlightGear1/2
  Angle Conversion/1 -> Selector/1
  Ground12/1 -> Flat Earth to LLA/2
  Compare To Zero/1 -> Stop Simulation/1
  Selector/1 -> Demux4/1
  Flat Earth to LLA/2 -> Compare To Zero/1, Pack net_fdm Packet for FlightGear1/3
  Bias2/1 -> Pack net_fdm Packet for FlightGear1/6
  Ground18/1 -> Pack net_fdm Packet for FlightGear1/33
  Ground20/1 -> Pack net_fdm Packet for FlightGear1/35
  Ground13/1 -> Pack net_fdm Packet for FlightGear1/36
  Ground16/1 -> Pack net_fdm Packet for FlightGear1/31
  Ground14/1 -> Pack net_fdm Packet for FlightGear1/37
  Ground15/1 -> Pack net_fdm Packet for FlightGear1/30
  Ground19/1 -> Pack net_fdm Packet for FlightGear1/34
  Ground17/1 -> Pack net_fdm Packet for FlightGear1/32
  Ground24/1 -> Pack net_fdm Packet for FlightGear1/28
  Constant1/1 -> Pack net_fdm Packet for FlightGear1/26
  Constant/1 -> Pack net_fdm Packet for FlightGear1/25
  Ground25/1 -> Pack net_fdm Packet for FlightGear1/29
  Connect to enable rotor animation/1 -> Pack net_fdm Packet for FlightGear1/27
  delta/1 -> Connect to enable rotor animation/1
  Length Conversion/1 -> Pack net_fdm Packet for FlightGear1/14
  Length Conversion1/1 -> Pack net_fdm Packet for FlightGear1/15
  Length Conversion2/1 -> Pack net_fdm Packet for FlightGear1/16
  V_e/1 -> cast12/1
  X_body/1 -> Flat Earth to LLA/1

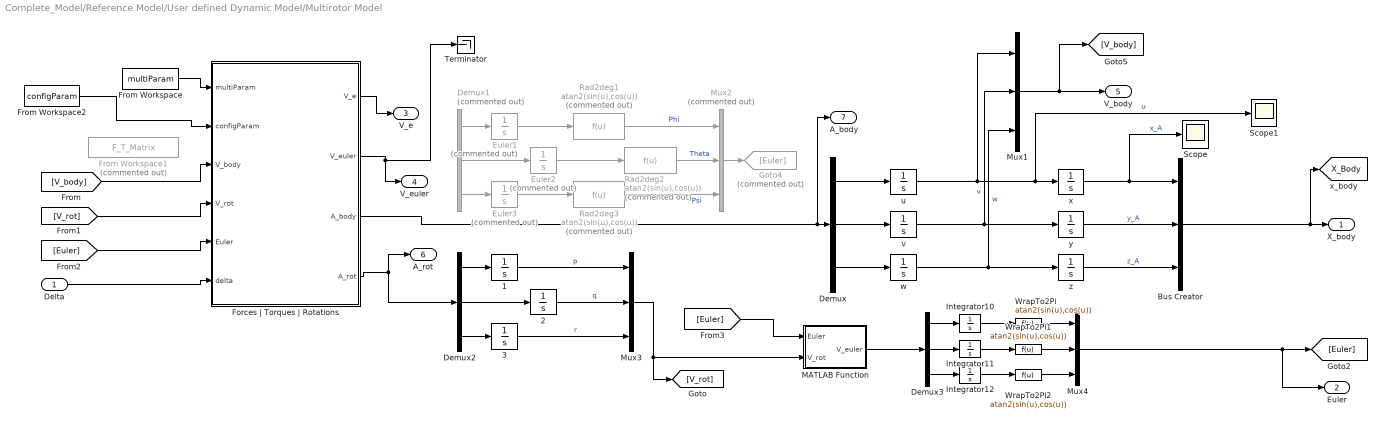
== system Complete_Model/Reference Model/User defined Dynamic Model/Multirotor Model  ==
  "Delta " : Inport
  1 : Integrator
  2 : Integrator
  3 : Integrator
  Bus Creator : BusCreator  Inputs=3
  Demux : Demux  Outputs=3
  Demux1 : Demux  Commented=on  Outputs=3
  Demux2 : Demux  Outputs=3
  Demux3 : Demux  Outputs=3
  Euler1 : Integrator  Commented=on
  Euler2 : Integrator  Commented=on
  Euler3 : Integrator  Commented=on
  Forces | Torques | Rotations : MATLAB Function  TreatAsAtomicUnit=on
  From Workspace : FromWorkspace  VariableName=multiParam  SampleTime=0
  From Workspace1 : FromWorkspace  Commented=on  VariableName=F_T_Matrix  SampleTime=0
  From Workspace2 : FromWorkspace  VariableName=configParam  SampleTime=0
  Goto4 : Goto  Commented=on  GotoTag=Euler
  Integrator10 : Integrator
  Integrator11 : Integrator
  Integrator12 : Integrator
  MATLAB Function : MATLAB Function  TreatAsAtomicUnit=on
  Mux1 : Mux  Inputs=3
  Mux2 : Mux  Commented=on  Inputs=3
  Mux3 : Mux  Inputs=3
  Mux4 : Mux  Inputs=[1;1;1]
  Rad2deg1 : Fcn  Commented=on  Expr=atan2(sin(u),cos(u))
  Rad2deg2 : Fcn  Commented=on  Expr=atan2(sin(u),cos(u))
  Rad2deg3 : Fcn  Commented=on  Expr=atan2(sin(u),cos(u))
  Scope : Scope
      settings: YMin=-1e-05  YMax=0.00012  SaveName=ScopeData10
  Scope1 : Scope
      settings: YMin=-15  YMax=17.5  SaveName=ScopeData11
  Terminator : Terminator
  WrapTo2Pi : Fcn  Expr=atan2(sin(u),cos(u))
  WrapTo2Pi1 : Fcn  Expr=atan2(sin(u),cos(u))
  WrapTo2Pi2 : Fcn  Expr=atan2(sin(u),cos(u))
  u : Integrator
  v : Integrator
  w : Integrator
  x : Integrator
  y : Integrator
  z : Integrator
  X_body : Outport
  Euler : Outport  Port=2
  V_e : Outport  Port=3
  V_euler : Outport  Port=4
  V_body : Outport  Port=5
  A_rot : Outport  Port=6
  A_body : Outport  Port=7
  tag scope: X_Body=global
  wires:
  Forces | Torques | Rotations/3(A_body) -> A_body/1, Demux/1
  [Euler] -> Forces | Torques | Rotations/5(Euler)
  Forces | Torques | Rotations/1(V_e) -> V_e/1
  Demux/3 -> w/1
  x/1 -> Scope/1, Bus Creator/1  "x_A"
  Demux/1 -> u/1
  w/1 -> Mux1/3, z/1  "w"
  [V_body] -> Forces | Torques | Rotations/3(V_body)
  z/1 -> Bus Creator/3  "z_A"
  Demux/2 -> v/1
  v/1 -> Mux1/2, y/1  "v"
  From Workspace/1 -> Forces | Torques | Rotations/1(multiParam)
  "Delta "/1 -> Forces | Torques | Rotations/6(delta)
  y/1 -> Bus Creator/2  "y_A"
  u/1 -> Mux1/1, Scope1/1, x/1  "u"
  Forces | Torques | Rotations/2(V_euler) -> Terminator/1, V_euler/1
  Mux1/1 -> [V_body], V_body/1
  Demux1/1 -> Euler1/1
  Demux1/2 -> Euler2/1
  Demux1/3 -> Euler3/1
  Euler1/1 -> Rad2deg1/1
  Euler2/1 -> Rad2deg2/1
  Euler3/1 -> Rad2deg3/1
  Rad2deg1/1 -> Mux2/1  "Phi"
  Rad2deg2/1 -> Mux2/2  "Theta"
  Rad2deg3/1 -> Mux2/3  "Psi"
  Mux2/1 -> Goto4/1
  Demux2/1 -> 1/1
  Demux2/2 -> 2/1
  Demux2/3 -> 3/1
  1/1 -> Mux3/1  "p"
  2/1 -> Mux3/2  "q"
  3/1 -> Mux3/3  "r"
  [V_rot] -> Forces | Torques | Rotations/4(V_rot)
  Mux3/1 -> MATLAB Function/2(V_rot), [V_rot]
  [Euler] -> MATLAB Function/1(Euler)
  Demux3/2 -> Integrator11/1
  Demux3/1 -> Integrator10/1
  Demux3/3 -> Integrator12/1
  Integrator10/1 -> WrapTo2Pi/1
  Integrator11/1 -> WrapTo2Pi1/1
  Integrator12/1 -> WrapTo2Pi2/1
  WrapTo2Pi/1 -> Mux4/1
  WrapTo2Pi1/1 -> Mux4/2
  WrapTo2Pi2/1 -> Mux4/3
  From Workspace2/1 -> Forces | Torques | Rotations/2(configParam)
  Bus Creator/1 -> [X_Body], X_body/1
  Mux4/1 -> Euler/1, [Euler]
  MATLAB Function/1(V_euler) -> Demux3/1
  Forces | Torques | Rotations/4(A_rot) -> Demux2/1, A_rot/1

== matlab function Complete_Model/Attitude//Position Control/Generate PWM Signals ==
  data: delta output; multiParam input; configParam input; F_T_Matrix parameter; F input; t_Phi input; t_Theta input; t_Psi input; Fxyz output; Mxyz output
function [delta, Fxyz, Mxyz]  = PWMgen (multiParam, configParam, F_T_Matrix, F, t_Phi, t_Theta, t_Psi) 

Mass = multiParam(1);               % multiParam defined in Run_First
Ixx = multiParam(2);
Iyy = multiParam(3);
Izz = multiParam(4);
k1 = multiParam(5);
k2 = multiParam(6);
l = multiParam(7);
g = multiParam(8);
configNum = configParam(1);
configOrient = configParam(2);
   
ForceTorque = [F,t_Phi, t_Theta, t_Psi]';
Fxyz = ForceTorque(1);
Mxyz = ForceTorque(2:4);

delta = F_T_Matrix*ForceTorque;     % Compute motor control signals "delta"

== matlab function Complete_Model/Reference Model/User defined Dynamic Model/Multirotor Model /Forces | Torques | Rotations ==
  data: multiParam input; configParam input; F_T_Matrix parameter; V_e output; V_body input size=3; V_rot input size=3; Euler input; delta input; V_euler output; A_body output; A_rot output
function [V_e, V_euler, A_body, A_rot] = Model(multiParam, configParam, F_T_Matrix, V_body, V_rot, Euler, delta)

% Created by Bryce Hill 7/7/14

% Function provides motor force and torque as well as state information and
% converts sensor data to North East Down (NED) and Global Coortinate
% Systems (GCS) 

% Call Values from Run_First | This way you should only need to edit the
% physical parameters of the multirotor one time in Run_First

% Variable calls and definitions ==========================================
Mass = multiParam(1);           % multiParam defined in Run_First
Ixx = multiParam(2);
Iyy = multiParam(3);
Izz = multiParam(4);
k1 = multiParam(5);
k2 = multiParam(6);
l = multiParam(7);
g = multiParam(8);
configNum = configParam(1);

MotorForceTorque = F_T_Matrix; % to bring in a matrix from the workspace 
                               % you must, from this window go to "Edit data", 
                               % select the variable, and change "scope" to "parameter"

p = V_rot(1);                   % V_rot defined in/by
q = V_rot(2);
r = V_rot(3);

u = V_body(1);                  % V_body defined in/by
v = V_body(2);
w = V_body(3);

Phi = Euler(1);                 % Euler defined in/by
Theta = Euler(2);
Psi = Euler(3);

% For ease of matrix definitions:
cPhi = cos(Phi);        sPhi = sin(Phi);        tPhi = tan(Phi);
cTheta = cos(Theta);    sTheta = sin(Theta);    tTheta = tan(Theta);
cPsi = cos(Psi);        sPsi = sin(Psi);        tPsi = tan(Psi);

%% Forces & Torques generated by motors ===================================

ForceTorque = MotorForceTorque*delta;                                                   
% Fx = ForceTorque(1);                        % Should be = 0 (Fixed motors)
% Fy = ForceTorque(2);                        % Should be = 0 (Fixed motors)
Fz = ForceTorque(1);                        
t_phi = ForceTorque(2);
t_theta = ForceTorque(3);
t_psi = ForceTorque(4);

%% Velocities =============================================================

% Inertial/Navigation (Global) (Pn_dot, Pe_dot & h_dot)
Vbody2Inertial = [cTheta*cPsi sPhi*sTheta*cPsi-cPhi*sPsi cPhi*sTheta*cPsi+sPhi*sPsi
                  cTheta*sPsi sPhi*sTheta*sPsi+cPhi*cPsi cPhi*sTheta*sPsi-sPhi*cPsi
                  sTheta -sPhi*cTheta -cPhi*cTheta];

V_e = Vbody2Inertial*V_body;        % nomenclature defines V_inertial as = V_e

% Body rotational rates 2 euler rates [(p q r) -> (phi_dot theta_dot
% psi_dot) | m/s
body2euler = [1 sPhi*tTheta cPsi*tTheta
              0 cPhi        -sPhi      
              0 sPhi/cTheta cPhi/cTheta];

V_euler = body2euler*V_rot;

%% Accelerations ==========================================================

% Body acceleration (u_dot v_dot w_dot) | (m/s^2)
A_body = [r*v-q*w-g*sTheta
          p*w-r*u+g*cTheta*sPhi
          q*u-p*v+g*cTheta*cPhi-Fz/Mass];

% Rotational Acceleration-Body Coordinates(p_dot q_dot r_dot) | m/s^2
A_rot = [(Iyy-Izz)/Ixx*q*r+t_phi/Ixx
         (Izz-Ixx)/Iyy*p*r+t_theta
         (Ixx-Iyy)/Izz*p*q+t_psi/Izz];

== matlab function Complete_Model/Attitude//Position Control/Attitude//Accel Control  ==
  data: multiParam input; PIDcmd output; A_body input; Euler input; A_cmd input; PIDerror output
function [PIDcmd,PIDerror]= PID(multiParam,A_body,Euler,A_cmd)
%#codegen

g = 9.71;%multiParam(8);       
Mass = 2.4;%multiParam(1);
Phi = Euler(1);
Theta = Euler(2);
Psi = Euler(3);
% Command accelerations 
ux = A_cmd(1);
uy = A_cmd(2);
uz = A_cmd(3);
% Measured (Body Frame Coordinates) accelerations from on board sensors
Ax = A_body(1);
Ay = A_body(2);
Az = A_body(3);


cPh = cos(Phi);     sPh = sin(Phi);
cTh = cos(Theta);   sTh = sin(Theta);
cPs = cos(Psi);     sPs = sin(Psi);

% Body2InertialR = [  cTh     sPh*sTh     cPh*sTh
%                     0       cPh         -sPh
%                    -sTh     sPh*cTh     cPh*cTh];

               
% Aned = Body2InertialR*[Ax Ay Az]';

F = Mass*((g-uz)/(cos(Phi)*cos(Theta)));    % Commanded Force Input (Beard 2008,40) 
Phicmd = atan((uy*cos(Theta))/(g-uz));      % Commanded Phi (roll) angle (Beard 2008,40)
Thetacmd = atan(ux/(uz-g));                 % Commanded Theta (pitch) angle (Beard 2008,40)
Psicmd = 0;                                 % Commanded Psi (yaw) angle = 0 why?

PIDcmd = [F Phicmd Thetacmd Psicmd]';
PIDerror = [uz-Az Phicmd-Phi Thetacmd-Theta Psicmd-Psi]';     
% PIDerror = [F-Mass*((g-Az)/(cos(Phi)*cos(Theta))) Phicmd-Phi Thetacmd-Theta Psicmd-Psi]';     


% Fcmd-Mass*((g-Az)/(cPhi*cTheta))

== matlab function Complete_Model/Reference Model/User defined Dynamic Model/Multirotor Model /MATLAB Function ==
  data: Euler input; V_euler output; V_rot input
function V_euler = fcn(Euler, V_rot)
%#codegen
Phi = Euler(1);                 % Euler defined in/by
Theta = Euler(2);
Psi = Euler(3);


Body2Euler = [1 sin(Phi)*tan(Theta) cos(Phi)*tan(Theta)
              0 cos(Phi)                       -sin(Phi)
              0 sin(Phi)/cos(Theta)            cos(Phi)/cos(Theta)           ];
          
V_euler = Body2Euler*V_rot;

== matlab function Complete_Model/Attitude//Position Control/Actuator Allocation ==
  data: multiParam input; delta input; M1 output; M2 output; M3 output; M4 output; M5 output; M6 output
function [M1, M2, M3, M4, M5, M6] = Control_Allocation(multiParam,delta)

% Select necessary values from multiParam

k1 = multiParam(5);
k2 = multiParam(6);
l = multiParam(7);

% variables A & B are placeholders
if length(delta) > 4
    A = [1000*k1*delta(1)+1000           1000*k1*delta(2)+1000          1000*k1*delta(3)+1000              1000*k1*delta(4)+1000                1000*k1*delta(5)+1000            1000*k1*delta(6)+1000
         500*(-.5*l*k1)*delta(1)+1500    500*(-l*k1)*delta(2)+1500      500*(-.5*l*k1)*delta(3)+1500       500*(.5*l*k1)*delta(4)+1500          500*(l*k1)*delta(5)+1500         500*(5*l*k1)*delta(6)+1500
         500*sqrt(3)/2*l*k1*delta(1)+500 0*delta(2)                     -sqrt(3)/2*l*k1*500*delta(3)+1500  -sqrt(3)/2*l*k1*500*delta(4)+1500    0*delta(5)                       500*sqrt(3)/2*l*k1*delta(6)+1500
         -k2*500*delta(1)+1500           k2*500*delta(2)+1500           -k2*500*delta(3)+1500              k2*500*delta(4)+1500                 -k2*500*delta(5)+1500            k2*500*delta(6)+1500            ];

else %length(delta) = 4
    A = [1000*k1*delta(1)+1000           1000*k1*delta(2)+1000          1000*k1*delta(3)+1000              1000*k1*delta(4)+1000                
         500*(-.5*l*k1)*delta(1)+1500    500*(-l*k1)*delta(2)+1500      500*(-.5*l*k1)*delta(3)+1500       500*(.5*l*k1)*delta(4)+1500          
         500*sqrt(3)/2*l*k1*delta(1)+500 0*delta(2)                     -sqrt(3)/2*l*k1*500*delta(3)+1500  -sqrt(3)/2*l*k1*500*delta(4)+1500 
         -k2*500*delta(1)+1500           k2*500*delta(2)+1500           -k2*500*delta(3)+1500              k2*500*delta(4)+1500              ];
% A = [k1*delta(1)+1000           k1*delta(2)+1000          k1*delta(3)+1000              k1*delta(4)+1000                k1*delta(5)+1000            k1*delta(6)+1000
%      (-.5*l*k1)*delta(1)+1500    (-l*k1)*delta(2)+1500      (-.5*l*k1)*delta(3)+1500       (.5*l*k1)*delta(4)+1500          (l*k1)*delta(5)+1500         (5*l*k1)*delta(6)+1500
%      sqrt(3)/2*l*k1*delta(1)+500 0*delta(2)                     -sqrt(3)/2*l*k1*delta(3)+1500  -sqrt(3)/2*l*k1*delta(4)+1500    0*delta(5)                       sqrt(3)/2*l*k1*delta(6)+1500
%      -k2*delta(1)+1500           k2*delta(2)+1500           -k2*delta(3)+1500              k2*delta(4)+1500                 -k2*delta(5)+1500            k2*delta(6)+1500            ];

% B = delta*16.667+1000;
end

B = sum(A,1);

% Motor distribution. This is necessary because the paper "QuadRotor
% Reference Model" used a clockwise count to number the motors whereas the
% pixhawk recognizes different numbering scheme. 
    
if length(B) > 4
    M5 = B(1);
    M1 = B(2);
    M4 = B(3);
    M6 = B(4);
    M2 = B(5);
    M3 = B(6);
else
    M1 = B(1);
    M4 = B(2);
    M2 = B(3);
    M3 = B(4);
    M5 = 0;
    M6 = 0;
end

== matlab function Complete_Model/Command Accelerations/Waypoint Acceleration Generator1 ==
  data: Position_desired input; Accel_ERROR output; Pos_Actual input
function Accel_ERROR  = Waypoint2Accel_Command(Position_desired, Pos_Actual)
%#codegen

x_d = Position_desired(1);
y_d = Position_desired(2);
z_d = Position_desired(3);

x_A = Pos_Actual(1);
y_A = Pos_Actual(2);
z_A = Pos_Actual(3);



% if abs(x_d-x_A) <= 5
%     u_x = 1*((x_d-x_A)/x_d);
% else
%     u_x = 3;
% end
% 
% if abs(y_d-y_A) <= 5
%     u_y = 1*((y_d-y_A)/y_d);
% else
%     u_y = 3;
% end
% 
% if abs(z_d-z_A) <= 5
%     u_z = 1*((z_d-z_A)/z_d);
% else
%     u_z = 3;
% end

x_er = x_d-x_A;
y_er = y_d-y_A;
z_er = z_d-z_A;

Accel_ERROR = [x_er y_er z_er]';
